simulink model "allmodes_group11"  (R2023a)
settings: Solver=FixedStepAuto  StartTime=0.0  StopTime=10.0  FixedStep=1e-3  RelTol=1e-3  EnableMultiTasking=on
undefined symbols (not defined in the file): a, A0, A1, b, c, D0, D1, D10, D11, D12, D13, D2, D3, D4, D5, D6, D7, D8, D9, magnitude, PTA0, PTA1, PTA2, PTB2, PTB23, PTB3, PTB9, PTC16, PTC17, PTC2, PTC3, PTC4, PTD0, PTD1, PTD2, PTD3
libraries: etargetslib x22, frdmk64flib x19, simulink x2, hdlsllib x1, dspstat3 x1
settings Model: ExtModeTrigDuration=5  Creator=faraa  LastModifiedBy=faraa
settings OptimizationCC: EnhancedBackFolding=on  PassReuseOutputArgsAs=Individual arguments  ZeroExternalMemoryAtStartup=off  ZeroInternalMemoryAtStartup=off  MaxStackSize=64  OptimizeBlockOrder=speed  DifferentSizesBufferReuse=on  OptimizationCustomize=off  EfficientTunableParamExpr=on
settings DebuggingCC: ParameterTunabilityLossMsg=error
settings HardwareCC: ProdBitPerPointer=32  ProdBitPerSizeT=32  ProdBitPerPtrDiffT=32  ProdLargestAtomicInteger=Long  ProdLargestAtomicFloat=Double  ProdWordSize=32  ProdHWDeviceType=ARM Compatible->ARM Cortex
settings SFSimCC: MATLABDynamicMemAlloc=off
settings RTWCC: Description=Embedded Coder  SystemTargetFile=ert.tlc  HardwareBoard=NXP FRDM-K64F  TLCOptions="-aInlineSetEventsForThisBaseRateFcn=TLC_FALSE -aSuppressMultiTaskScheduler=TLC_FALSE  -aRateBasedStepFcn=0"  TemplateMakefile=ert_default_tmf  Toolchain=GNU Tools for ARM Embedded Processors
settings CodeAppCC: ForceParamTrailComments=on  IgnoreCustomStorageClasses=off  OperatorAnnotations=on  SimulinkDataObjDesc=on  SFDataObjDesc=on  InsertBlockDesc=on
settings ERTTargetCC: ExtModeTransport=4  ExtModeMexFile=sendToCommService

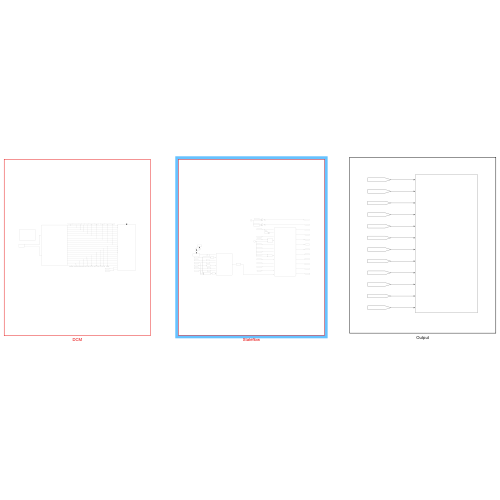
[thumbnail: Simulink's stored preview of the top-level diagram]
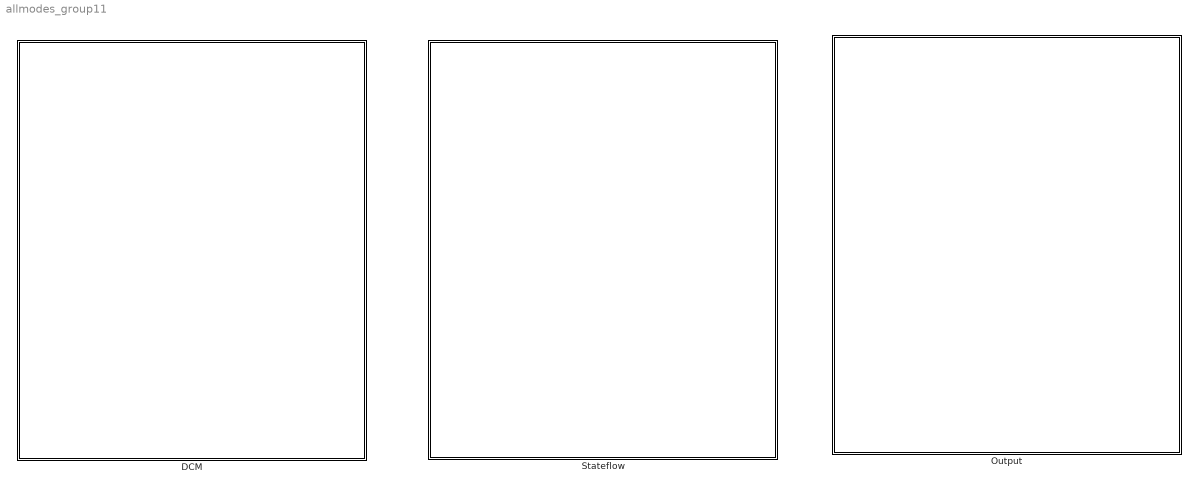
== system allmodes_group11 ==
  DCM : Subsystem
  Output : Subsystem
  Stateflow : Subsystem

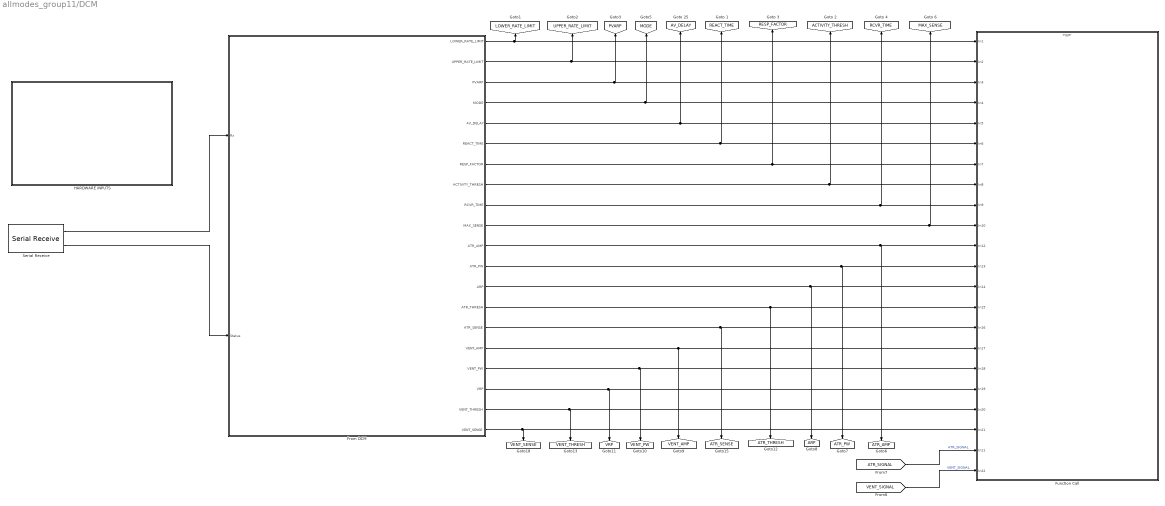
== system allmodes_group11/DCM ==
  From DCM : Stateflow chart  TreatAsAtomicUnit=on
  Function Call : Subsystem  TreatAsAtomicUnit=on
  HARDWARE INPUTS : Subsystem
  Serial Receive : frdmk64flib/Serial Receive  SCIModule=0  Baudrate=uint32(9600)  Parity=None  StopBits=1  HardwareFlowControl=None  ByteOrder=LittleEndian  DataType=uint8  DataLength=86  BlockingMode=off  OutputStatus=on  SampleTime=-1
  tag scope: ACTIVITY_THRESH=global, ARP=global, ATR_AMP=global, ATR_PW=global, ATR_SENSE=global, ATR_THRESH=global, AV_DELAY=global, LOWER_RATE_LIMIT=global, MAX_SENSE=global, MODE=global, PVARP=global, RCVR_TIME=global, REACT_TIME=global, RESP_FACTOR=global, UPPER_RATE_LIMIT=global, VENT_AMP=global, VENT_PW=global, VENT_SENSE=global, VENT_THRESH=global, VRP=global
  wires:
  Serial Receive/1 -> From DCM/1(Rx)
  Serial Receive/2 -> From DCM/2(Status)
  From DCM/1(LOWER_RATE_LIMIT) -> Function Call/1(In1), [LOWER_RATE_LIMIT]
  From DCM/2(UPPER_RATE_LIMIT) -> Function Call/2(In2), [UPPER_RATE_LIMIT]
  From DCM/3(PVARP) -> [PVARP], Function Call/3(In3)
  From DCM/4(MODE) -> Function Call/4(In4), [MODE]
  From DCM/5(AV_DELAY) -> [AV_DELAY], Function Call/5(In5)
  From DCM/6(REACT_TIME) -> Function Call/6(In6), [REACT_TIME]
  From DCM/7(RESP_FACTOR) -> [RESP_FACTOR], Function Call/7(In7)
  From DCM/8(ACTIVITY_THRESH) -> [ACTIVITY_THRESH], Function Call/8(In8)
  From DCM/9(RCVR_TIME) -> [RCVR_TIME], Function Call/9(In9)
  From DCM/10(MAX_SENSE) -> [MAX_SENSE], Function Call/10(In10)
  From DCM/11(ATR_AMP) -> Function Call/11(In12), [ATR_AMP]
  From DCM/12(ATR_PW) -> Function Call/12(In13), [ATR_PW]
  From DCM/13(ARP) -> Function Call/13(In14), [ARP]
  From DCM/14(ATR_THRESH) -> Function Call/14(In15), [ATR_THRESH]
  From DCM/15(ATR_SENSE) -> Function Call/15(In16), [ATR_SENSE]
  From DCM/16(VENT_AMP) -> Function Call/16(In17), [VENT_AMP]
  From DCM/17(VENT_PW) -> Function Call/17(In18), [VENT_PW]
  From DCM/18(VRP) -> Function Call/18(In19), [VRP]
  From DCM/19(VENT_THRESH) -> Function Call/19(In20), [VENT_THRESH]
  From DCM/20(VENT_SENSE) -> Function Call/20(In21), [VENT_SENSE]
  [ATR_SIGNAL] -> Function Call/21(In11)  "ATR_SIGNAL"
  [VENT_SIGNAL] -> Function Call/22(In22)  "VENT_SIGNAL"

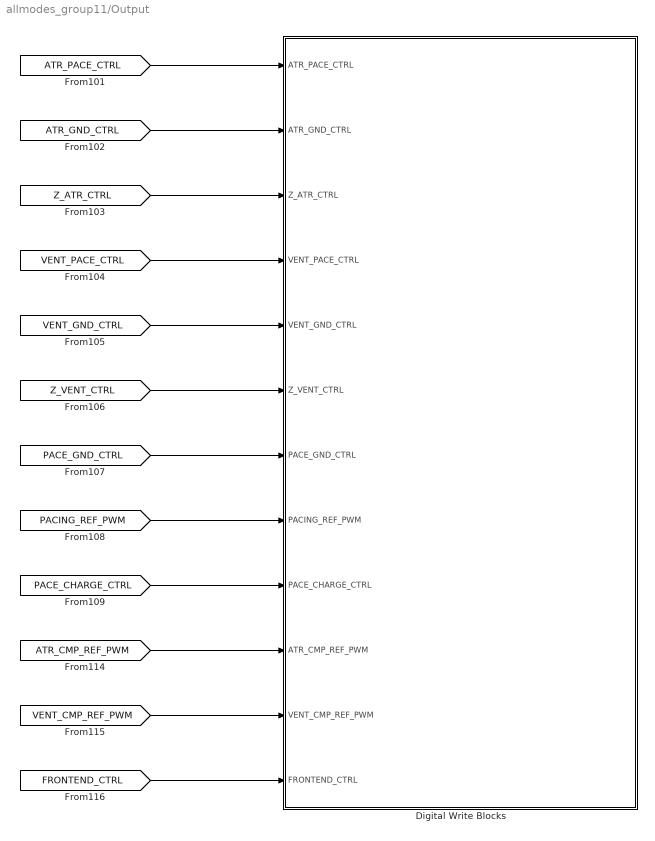
== system allmodes_group11/Output ==
  Digital Write Blocks : Subsystem
  wires:
  [Z_VENT_CTRL] -> Digital Write Blocks/6(Z_VENT_CTRL)
  [PACE_GND_CTRL] -> Digital Write Blocks/7(PACE_GND_CTRL)
  [ATR_PACE_CTRL] -> Digital Write Blocks/1(ATR_PACE_CTRL)
  [PACING_REF_PWM] -> Digital Write Blocks/8(PACING_REF_PWM)
  [VENT_GND_CTRL] -> Digital Write Blocks/5(VENT_GND_CTRL)
  [VENT_CMP_REF_PWM] -> Digital Write Blocks/11(VENT_CMP_REF_PWM)
  [PACE_CHARGE_CTRL] -> Digital Write Blocks/9(PACE_CHARGE_CTRL)
  [ATR_GND_CTRL] -> Digital Write Blocks/2(ATR_GND_CTRL)
  [VENT_PACE_CTRL] -> Digital Write Blocks/4(VENT_PACE_CTRL)
  [ATR_CMP_REF_PWM] -> Digital Write Blocks/10(ATR_CMP_REF_PWM)
  [Z_ATR_CTRL] -> Digital Write Blocks/3(Z_ATR_CTRL)
  [FRONTEND_CTRL] -> Digital Write Blocks/12(FRONTEND_CTRL)

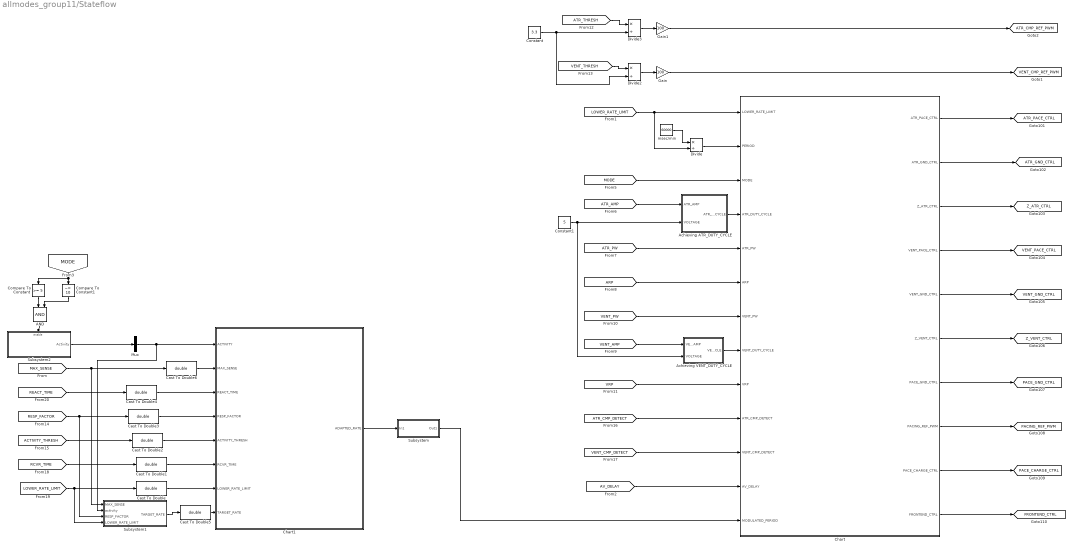
== system allmodes_group11/Stateflow ==
  AND : Logic  IconShape=distinctive  AllPortsSameDT=off  OutDataTypeStr=boolean
  Achieving ATR_DUTY_CYCLE : Subsystem
  Achieving VENT_DUTY_CYCLE : Subsystem
  Cast To Double{,1..6} (7 alike) : DataTypeConversion  OutDataTypeStr=double  SaturateOnIntegerOverflow=off  RndMeth=Floor
  Chart : Stateflow chart  TreatAsAtomicUnit=on
  Chart1 : Stateflow chart  TreatAsAtomicUnit=on
  Compare To Constant : simulink/Logic and Bit Operations/Compare To Constant  relop=>=  const=5  OutDataTypeStr=boolean
  Compare To Constant1 : simulink/Logic and Bit Operations/Compare To Constant  relop=~=  const=10  OutDataTypeStr=boolean
  Constant : Constant  Value=3.3
  Constant1 : Constant  Value=5
  Divide : Product  Inputs=*/
  Divide2 : Product  Inputs=*/
  Divide3 : Product  Inputs=*/
  Gain : Gain  Gain=100
  Gain1 : Gain  Gain=100
  Mux : Mux  Inputs=1
  Subsystem : Subsystem
  Subsystem1 : Subsystem
  Subsystem2 : Subsystem
  msec/min : Constant  Value=60000  OutDataTypeStr=double  LockScale=on
  tag scope: ATR_CMP_REF_PWM=global, ATR_GND_CTRL=global, ATR_PACE_CTRL=global, FRONTEND_CTRL=global, PACE_CHARGE_CTRL=global, PACE_GND_CTRL=global, PACING_REF_PWM=global, VENT_CMP_REF_PWM=global, VENT_GND_CTRL=global, VENT_PACE_CTRL=global, Z_ATR_CTRL=global, Z_VENT_CTRL=global
  wires:
  [VRP] -> Chart/9(VRP)
  [MODE] -> Chart/3(MODE)
  [LOWER_RATE_LIMIT] -> Divide/2, Chart/1(LOWER_RATE_LIMIT)
  [ATR_PW] -> Chart/5(ATR_PW)
  [ARP] -> Chart/6(ARP)
  [ATR_AMP] -> Achieving ATR_DUTY_CYCLE/1(ATR_AMP)
  Achieving ATR_DUTY_CYCLE/1(ATR_DUTY_CYCLE) -> Chart/4(ATR_DUTY_CYCLE)
  [VENT_PW] -> Chart/7(VENT_PW)
  [VENT_AMP] -> Achieving VENT_DUTY_CYCLE/1(VENT_AMP)
  Achieving VENT_DUTY_CYCLE/1(VENT_DUTY_CYCLE) -> Chart/8(VENT_DUTY_CYCLE)
  Chart/1(ATR_PACE_CTRL) -> [ATR_PACE_CTRL]
  Chart/2(ATR_GND_CTRL) -> [ATR_GND_CTRL]
  Chart/3(Z_ATR_CTRL) -> [Z_ATR_CTRL]
  Chart/4(VENT_PACE_CTRL) -> [VENT_PACE_CTRL]
  Chart/5(VENT_GND_CTRL) -> [VENT_GND_CTRL]
  Chart/6(Z_VENT_CTRL) -> [Z_VENT_CTRL]
  Chart/7(PACE_GND_CTRL) -> [PACE_GND_CTRL]
  Chart/8(PACING_REF_PWM) -> [PACING_REF_PWM]
  Chart/9(PACE_CHARGE_CTRL) -> [PACE_CHARGE_CTRL]
  Constant1/1 -> Achieving VENT_DUTY_CYCLE/2(VOLTAGE), Achieving ATR_DUTY_CYCLE/2(VOLTAGE)
  [ATR_CMP_DETECT] -> Chart/10(ATR_CMP_DETECT)
  [VENT_CMP_DETECT] -> Chart/11(VENT_CMP_DETECT)
  Divide/1 -> Chart/2(PERIOD)
  msec/min/1 -> Divide/1
  Chart/10(FRONTEND_CTRL) -> [FRONTEND_CTRL]
  Constant/1 -> Divide3/2, Divide2/2
  [ATR_THRESH] -> Divide3/1
  [VENT_THRESH] -> Divide2/1
  [AV_DELAY] -> Chart/12(AV_DELAY)
  Divide2/1 -> Gain/1
  Gain/1 -> [VENT_CMP_REF_PWM]
  Divide3/1 -> Gain1/1
  Gain1/1 -> [ATR_CMP_REF_PWM]
  [REACT_TIME] -> Cast To Double4/1
  [ACTIVITY_THRESH] -> Cast To Double2/1
  [LOWER_RATE_LIMIT] -> Cast To Double/1, Subsystem1/4(LOWER_RATE_LIMIT)
  [RCVR_TIME] -> Cast To Double1/1
  [MAX_SENSE] -> Cast To Double6/1, Subsystem1/1(MAX_SENSE)
  [MODE] -> Compare To Constant/1, Compare To Constant1/1
  [RESP_FACTOR] -> Subsystem1/3(RESP_FACTOR), Cast To Double3/1
  Subsystem2/1(Activity) -> Mux/1
  Subsystem/1(Out1) -> Chart/13(MODULATED_PERIOD)
  Compare To Constant/1 -> AND/1
  AND/1 -> Subsystem2/Enable
  Compare To Constant1/1 -> AND/2
  Subsystem1/1(TARGET_RATE) -> Cast To Double5/1
  Chart1/1(ADAPTED_RATE) -> Subsystem/1(In1)
  Mux/1 -> Subsystem1/2(activity), Chart1/1(ACTIVITY)
  Cast To Double/1 -> Chart1/7(LOWER_RATE_LIMIT)
  Cast To Double1/1 -> Chart1/6(RCVR_TIME)
  Cast To Double2/1 -> Chart1/5(ACTIVITY_THRESH)
  Cast To Double3/1 -> Chart1/4(RESP_FACTOR)
  Cast To Double4/1 -> Chart1/3(REACT_TIME)
  Cast To Double5/1 -> Chart1/8(TARGET_RATE)
  Cast To Double6/1 -> Chart1/2(MAX_SENSE)

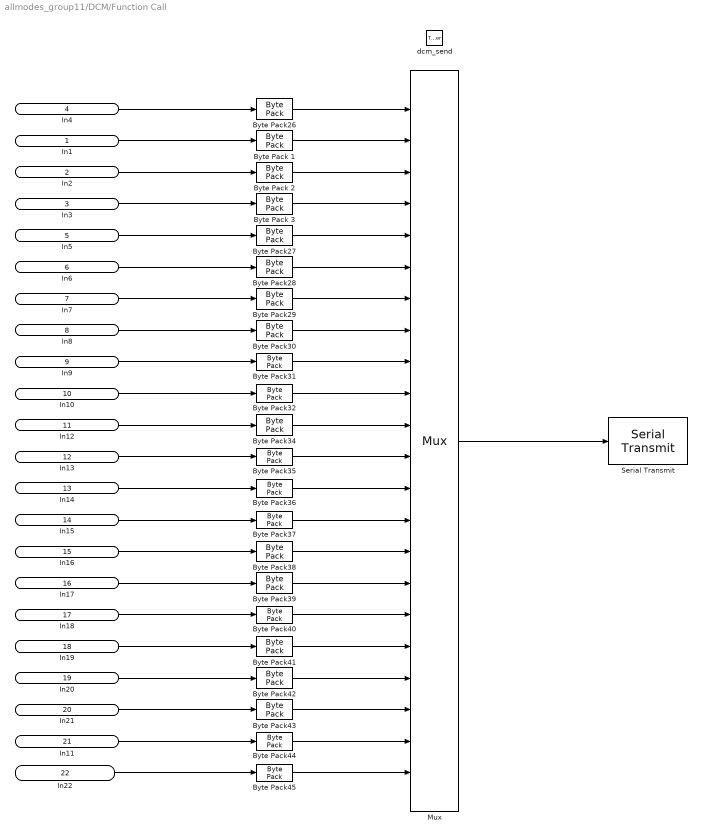
== system allmodes_group11/DCM/Function Call ==
  In1 : Inport
  In2 : Inport  Port=2
  In3 : Inport  Port=3
  In4 : Inport  Port=4
  In5 : Inport  Port=5
  In6 : Inport  Port=6
  In7 : Inport  Port=7
  In8 : Inport  Port=8
  In9 : Inport  Port=9
  In10 : Inport  Port=10
  In12 : Inport  Port=11
  In13 : Inport  Port=12
  In14 : Inport  Port=13
  In15 : Inport  Port=14
  In16 : Inport  Port=15
  In17 : Inport  Port=16
  In18 : Inport  Port=17
  In19 : Inport  Port=18
  In20 : Inport  Port=19
  In21 : Inport  Port=20
  In11 : Inport  Port=21
  In22 : Inport  Port=22
  dcm_send : TriggerPort  TriggerType=function-call  IsSimulinkFunction=on  FunctionName=dcm_send  VariantControl=Variant
  Byte Pack 1 : etargetslib/Byte Pack  datatypes={'uint16'}  byteAlign=1
  Byte Pack 2 : etargetslib/Byte Pack  datatypes={'uint16'}  byteAlign=1
  Byte Pack 3 : etargetslib/Byte Pack  datatypes={'uint16'}  byteAlign=1
  Byte Pack{26..29,31..32,35..36,40..41} (10 alike) : etargetslib/Byte Pack  datatypes={'uint16'}  byteAlign=1
  Byte Pack{30,34,37..39,42..45} (9 alike) : etargetslib/Byte Pack  datatypes={'double'}  byteAlign=1
  Mux : Mux  Inputs=22
  Serial Transmit : frdmk64flib/Serial Transmit  SCIModule=0  Baudrate=uint32(9600)  Parity=None  StopBits=1  HardwareFlowControl=None  ByteOrder=LittleEndian  BlockingMode=on  OutputStatus=on
  wires:
  In1/1 -> Byte Pack 1/1
  In2/1 -> Byte Pack 2/1
  In3/1 -> Byte Pack 3/1
  In4/1 -> Byte Pack26/1
  In5/1 -> Byte Pack27/1
  In6/1 -> Byte Pack28/1
  In7/1 -> Byte Pack29/1
  In8/1 -> Byte Pack30/1
  In9/1 -> Byte Pack31/1
  In10/1 -> Byte Pack32/1
  In12/1 -> Byte Pack34/1
  In13/1 -> Byte Pack35/1
  In14/1 -> Byte Pack36/1
  In15/1 -> Byte Pack37/1
  In16/1 -> Byte Pack38/1
  In17/1 -> Byte Pack39/1
  In18/1 -> Byte Pack40/1
  In19/1 -> Byte Pack41/1
  In20/1 -> Byte Pack42/1
  In21/1 -> Byte Pack43/1
  Byte Pack27/1 -> Mux/5
  Byte Pack28/1 -> Mux/6
  Byte Pack29/1 -> Mux/7
  Byte Pack30/1 -> Mux/8
  Byte Pack31/1 -> Mux/9
  Byte Pack32/1 -> Mux/10
  Byte Pack34/1 -> Mux/11
  Byte Pack35/1 -> Mux/12
  Byte Pack36/1 -> Mux/13
  Byte Pack37/1 -> Mux/14
  Byte Pack38/1 -> Mux/15
  Byte Pack39/1 -> Mux/16
  Byte Pack40/1 -> Mux/17
  Byte Pack41/1 -> Mux/18
  Byte Pack42/1 -> Mux/19
  Byte Pack43/1 -> Mux/20
  Mux/1 -> Serial Transmit/1
  Byte Pack44/1 -> Mux/21
  Byte Pack45/1 -> Mux/22
  Byte Pack26/1 -> Mux/1
  Byte Pack 1/1 -> Mux/2
  Byte Pack 2/1 -> Mux/3
  Byte Pack 3/1 -> Mux/4
  In22/1 -> Byte Pack45/1
  In11/1 -> Byte Pack44/1

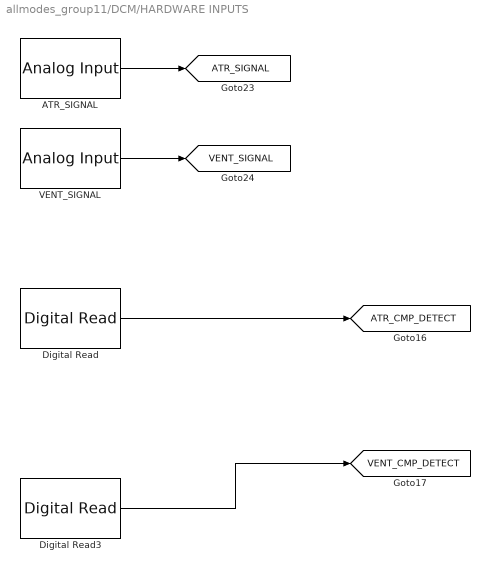
== system allmodes_group11/DCM/HARDWARE INPUTS ==
  ATR_SIGNAL : frdmk64flib/Analog Input  Whichpin=PTB2 (A0)  SampleTime=-1
  Digital Read : frdmk64flib/Digital Read  Whichpin=PTC16 (D0)  SampleTime=-1
  Digital Read3 : frdmk64flib/Digital Read  Whichpin=PTC17 (D1)  SampleTime=-1
  VENT_SIGNAL : frdmk64flib/Analog Input  Whichpin=PTB3 (A1)  SampleTime=-1
  tag scope: ATR_CMP_DETECT=global, ATR_SIGNAL=global, VENT_CMP_DETECT=global, VENT_SIGNAL=global
  wires:
  VENT_SIGNAL/1 -> [VENT_SIGNAL]
  ATR_SIGNAL/1 -> [ATR_SIGNAL]
  Digital Read3/1 -> [VENT_CMP_DETECT]
  Digital Read/1 -> [ATR_CMP_DETECT]

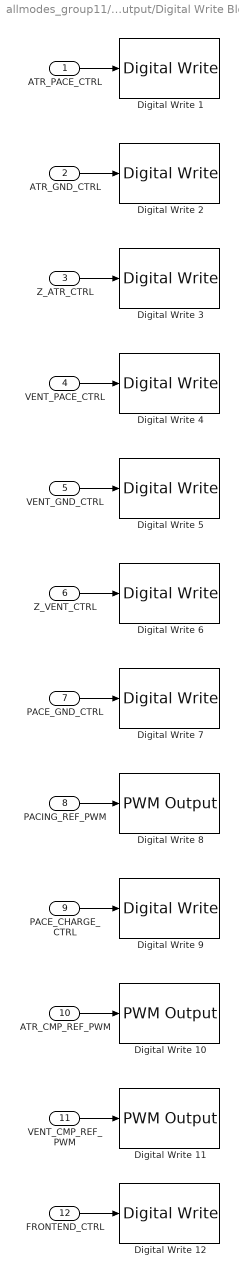
== system allmodes_group11/Output/Digital Write Blocks ==
  ATR_PACE_CTRL : Inport
  ATR_GND_CTRL : Inport  Port=2
  Z_ATR_CTRL : Inport  Port=3
  VENT_PACE_CTRL : Inport  Port=4
  VENT_GND_CTRL : Inport  Port=5
  Z_VENT_CTRL : Inport  Port=6
  PACE_GND_CTRL : Inport  Port=7
  PACING_REF_PWM : Inport  Port=8
  PACE_CHARGE_CTRL : Inport  Port=9
  ATR_CMP_REF_PWM : Inport  Port=10
  VENT_CMP_REF_PWM : Inport  Port=11  OutDataTypeStr=double
  FRONTEND_CTRL : Inport  Port=12
  Digital Write 1 : frdmk64flib/Digital Write  Whichpin=PTA0 (D8)
  Digital Write 10 : frdmk64flib/PWM Output  Whichpin=PTC2 (D6)  InitialFrequency=2000  InitialDutyCycle=30
  Digital Write 11 : frdmk64flib/PWM Output  Whichpin=PTA1 (D3)  InitialFrequency=2000  InitialDutyCycle=30
  Digital Write 12 : frdmk64flib/Digital Write  Whichpin=PTD1 (D13)
  Digital Write 2 : frdmk64flib/Digital Write  Whichpin=PTD2 (D11)
  Digital Write 3 : frdmk64flib/Digital Write  Whichpin=PTB23 (D4)
  Digital Write 4 : frdmk64flib/Digital Write  Whichpin=PTC4 (D9)
  Digital Write 5 : frdmk64flib/Digital Write  Whichpin=PTD3 (D12)
  Digital Write 6 : frdmk64flib/Digital Write  Whichpin=PTC3 (D7)
  Digital Write 7 : frdmk64flib/Digital Write  Whichpin=PTD0 (D10)
  Digital Write 8 : frdmk64flib/PWM Output  Whichpin=PTA2 (D5)  InitialFrequency=2000  InitialDutyCycle=30
  Digital Write 9 : frdmk64flib/Digital Write  Whichpin=PTB9 (D2)
  wires:
  VENT_PACE_CTRL/1 -> Digital Write 4/1
  VENT_GND_CTRL/1 -> Digital Write 5/1
  ATR_GND_CTRL/1 -> Digital Write 2/1
  PACING_REF_PWM/1 -> Digital Write 8/1
  ATR_PACE_CTRL/1 -> Digital Write 1/1
  PACE_GND_CTRL/1 -> Digital Write 7/1
  Z_VENT_CTRL/1 -> Digital Write 6/1
  PACE_CHARGE_CTRL/1 -> Digital Write 9/1
  Z_ATR_CTRL/1 -> Digital Write 3/1
  ATR_CMP_REF_PWM/1 -> Digital Write 10/1
  VENT_CMP_REF_PWM/1 -> Digital Write 11/1
  FRONTEND_CTRL/1 -> Digital Write 12/1

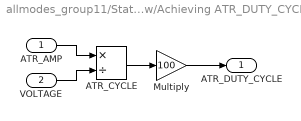
== system allmodes_group11/Stateflow/Achieving ATR_DUTY_CYCLE ==
  ATR_AMP : Inport
  VOLTAGE : Inport  Port=2
  ATR_CYCLE : Product  Inputs=*/
  Multiply : Gain  Gain=100
  ATR_DUTY_CYCLE : Outport  VectorParamsAs1DForOutWhenUnconnected=off
  wires:
  ATR_AMP/1 -> ATR_CYCLE/1
  VOLTAGE/1 -> ATR_CYCLE/2
  ATR_CYCLE/1 -> Multiply/1
  Multiply/1 -> ATR_DUTY_CYCLE/1

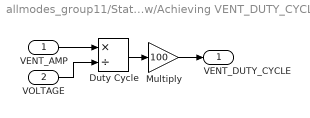
== system allmodes_group11/Stateflow/Achieving VENT_DUTY_CYCLE ==
  VENT_AMP : Inport
  VOLTAGE : Inport  Port=2
  Duty Cycle : Product  Inputs=*/
  Multiply : Gain  Gain=100
  VENT_DUTY_CYCLE : Outport  VectorParamsAs1DForOutWhenUnconnected=off
  wires:
  VENT_AMP/1 -> Duty Cycle/1
  VOLTAGE/1 -> Duty Cycle/2
  Duty Cycle/1 -> Multiply/1
  Multiply/1 -> VENT_DUTY_CYCLE/1

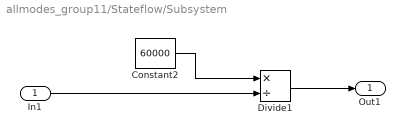
== system allmodes_group11/Stateflow/Subsystem ==
  In1 : Inport
  Constant2 : Constant  Value=60000
  Divide1 : Product  Inputs=*/
  Out1 : Outport
  wires:
  In1/1 -> Divide1/2
  Constant2/1 -> Divide1/1
  Divide1/1 -> Out1/1

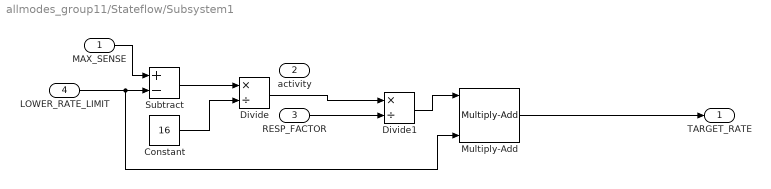
== system allmodes_group11/Stateflow/Subsystem1 ==
  MAX_SENSE : Inport
  activity : Inport  Port=2
  RESP_FACTOR : Inport  Port=3
  LOWER_RATE_LIMIT : Inport  Port=4
  Constant : Constant  Value=16
  Divide : Product  Inputs=*/
  Divide1 : Product  Inputs=*/
  Multiply-Add : hdlsllib/HDL Operations/Multiply-Add  Function=c+(a.*b)  datatype=uint16  RndMeth=Nearest  DoSatur=off  FMA=off
  Subtract : Sum  Inputs=+-
  TARGET_RATE : Outport  OutDataTypeStr=uint16  SourceOfInitialOutputValue=Input signal
  wires:
  MAX_SENSE/1 -> Subtract/1
  LOWER_RATE_LIMIT/1 -> Multiply-Add/3, Subtract/2
  Subtract/1 -> Divide/1
  Constant/1 -> Divide/2
  Divide/1 -> Divide1/1
  RESP_FACTOR/1 -> Divide1/2
  Divide1/1 -> Multiply-Add/1
  Multiply-Add/1 -> TARGET_RATE/1

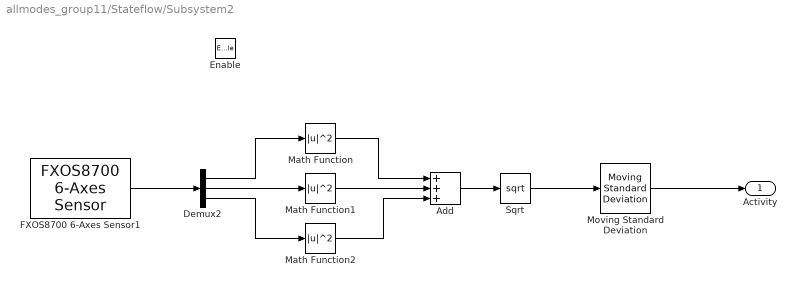
== system allmodes_group11/Stateflow/Subsystem2 ==
  Enable : EnablePort
  Add : Sum  Inputs=+++
  Demux2 : Demux  Outputs=3
  FXOS8700 6-Axes Sensor1 : frdmk64flib/FXOS8700 6-Axes Sensor  Activesensor=Accelerometer only  ODR=800Hz  HybridODR=400Hz  Accelfullrange=-4g to +4g  SampleTime=-1
  Math Function : Math  Operator=magnitude^2  SignedPower=on  OutDataTypeStr=double
  Math Function1 : Math  Operator=magnitude^2  SignedPower=on  OutDataTypeStr=double
  Math Function2 : Math  Operator=magnitude^2  SignedPower=on  OutDataTypeStr=double
  Moving Standard Deviation : dspstat3/Moving Standard Deviation  Method=Sliding window  ForgettingFactorPort=off  SpecifyWindowLength=on  WindowLength=128  OverlapLength=127  AllowArbitraryInputLength=off  ForgettingFactor=0.9  SimulateUsing=Code generation
  Sqrt : Sqrt
  Activity : Outport  SourceOfInitialOutputValue=Input signal
  wires:
  Sqrt/1 -> Moving Standard Deviation/1
  FXOS8700 6-Axes Sensor1/1 -> Demux2/1
  Math Function/1 -> Add/1
  Add/1 -> Sqrt/1
  Math Function2/1 -> Add/3
  Demux2/2 -> Math Function1/1
  Math Function1/1 -> Add/2
  Demux2/1 -> Math Function/1
  Demux2/3 -> Math Function2/1
  Moving Standard Deviation/1 -> Activity/1

== stateflow chart allmodes_group11/DCM/From DCM ==
  state ECHO_PARAM2
    entry:
    dcm_send();
  state Default
    %Setting values to variables if
    %not initialized in DCM
    entry:
    %GENERAL
    MODE = 7;
    LOWER_RATE_LIMIT = 60;
    UPPER_RATE_LIMIT = 120;
    PVARP = 250;
    AV_DELAY = 150;
    REACT_TIME = 50;
    RESP_FACTOR = 16;
    ACTIVITY_THRESH = 0.2;
    RCVR_TIME = 60;
    MAX_SENSE = 180;
    %ATRIUM
    ATR_AMP = 600;
    ATR_PW = 10;
    ARP = 200;
    ATR_THRESH = 1.8;
    ATR_SENSE = 800;
    %VENTRICLE
    VENT_AMP = 600;
    VENT_PW = 10;
    VRP = 200;
    VENT_THRESH = 2.2;
    VENT_SENSE = 800;
  state SET_PARAM
    entry:
    MODE = typecast(Rx(3:4), 'uint16');
    LOWER_RATE_LIMIT = typecast(Rx(5:6), 'uint16');
    UPPER_RATE_LIMIT = typecast(Rx(7:8), 'uint16');
    PVARP = typecast(Rx(9:10), 'uint16');
    AV_DELAY = typecast(Rx(11:12), 'uint16');
    REACT_TIME = typecast(Rx(13:14), 'uint16');
    RESP_FACTOR = typecast(Rx(15:16), 'uint16');
    ACTIVITY_THRESH = typecast(Rx(17:24), 'double');
    RCVR_TIME = typecast(Rx(25:26), 'uint16');
    MAX_SENSE = typecast(Rx(27:28), 'uint16');
    %ATR
    ATR_AMP = typecast(Rx(29:36), 'double');
    ATR_PW = typecast(Rx(37:38), 'uint16');
    ARP = typecast(Rx(39:40), 'uint16');
    ATR_THRESH = typecast(Rx(41:48), 'double');
    ATR_SENSE = typecast(Rx(49:56), 'double');
    %VENT
    VENT_AMP = typecast(Rx(57:64), 'double');
    VENT_PW = typecast(Rx(65:66), 'uint16');
    VRP = typecast(Rx(67:68), 'uint16');
    VENT_THRESH = typecast(Rx(69:76), 'double');
    VENT_SENSE = typecast(Rx(77:84), 'double');
  state STANDBY
  state ECHO_PARAM
    entry:
    dcm_send();
  ECHO_PARAM2 -> STANDBY
  SET_PARAM -> ECHO_PARAM2
  (default) -> Default
  (junction 7) -> STANDBY [order 2]
  Default -> STANDBY
  STANDBY -> (junction 7) : [Status == 0]
  (junction 7) -> (junction 10) [order 1] : [Rx(1) == hex2dec('00')]
  (junction 10) -> SET_PARAM [order 2] : [Rx(2) == hex2dec('00')]
  (junction 10) -> ECHO_PARAM [order 1] : [Rx(2) == hex2dec('01')]
  ECHO_PARAM -> STANDBY
  data: Rx input uint8; Status input uint8; LOWER_RATE_LIMIT output uint16; UPPER_RATE_LIMIT output uint16; PVARP output uint16; MODE output uint16; AV_DELAY output uint16; REACT_TIME output uint16; RESP_FACTOR output uint16; ACTIVITY_THRESH output double; RCVR_TIME output uint16; MAX_SENSE output uint16; ATR_AMP output double; ATR_PW output uint16; ARP output uint16; ATR_THRESH output double; ATR_SENSE output double; VENT_AMP output double; VENT_PW output uint16; VRP output uint16; VENT_THRESH output double; VENT_SENSE output double

== stateflow chart allmodes_group11/Stateflow/Chart ==
  state Start
  state AOO [group]
    state CHARGING
      during:
      %Begin Charging C22 Capacitor
      ATR_PACE_CTRL = LOW
      VENT_PACE_CTRL = LOW
      PACING_REF_PWM = ATR_DUTY_CYCLE
      PACE_CHARGE_CTRL = HIGH
      %Begin Discharging C21 Blocking Capacitor
      PACE_GND_CTRL = HIGH
      VENT_PACE_CTRL = LOW
      Z_ATR_CTRL = LOW
      Z_VENT_CTRL = LOW
      ATR_PACE_CTRL = LOW
      ATR_GND_CTRL = HIGH
      VENT_GND_CTRL = LOW
    state DISCHARGING
      during:
      %Discharge C22 into Atrium (AtrialPacing)
      %Begin Charging C21 Blocking Capacitor
      PACE_CHARGE_CTRL = LOW
      PACE_GND_CTRL = HIGH
      ATR_PACE_CTRL = HIGH
      ATR_GND_CTRL = LOW
      Z_ATR_CTRL = LOW
      Z_VENT_CTRL = LOW
      VENT_GND_CTRL = LOW
      VENT_PACE_CTRL  = LOW
    AOO.CHARGING -> AOO.DISCHARGING [order 1] : after(PERIOD-ATR_PW, msec)
    AOO.DISCHARGING -> AOO.CHARGING : after(ATR_PW, msec)
  state AAI [group]
    state PROXY
      during:
      %Discharge C21 Blocking Capacitor
      PACE_GND_CTRL = HIGH
      VENT_PACE_CTRL = LOW
      Z_ATR_CTRL = LOW
      Z_VENT_CTRL = LOW
      ATR_PACE_CTRL = LOW
      ATR_GND_CTRL = HIGH
      VENT_GND_CTRL = LOW
      %Charge C22
      ATR_PACE_CTRL = LOW
      VENT_PACE_CTRL = LOW
      PACING_REF_PWM = ATR_DUTY_CYCLE
      PACE_CHARGE_CTRL = HIGH
    state DISCHARGING
      during:
      %Discharge C22 into Atrium (Atrial Pacing)
      %Begin Charging Blocking Capacitor
      PACE_CHARGE_CTRL = LOW
      PACE_GND_CTRL = HIGH
      ATR_PACE_CTRL = HIGH
      ATR_GND_CTRL = LOW
      Z_ATR_CTRL = LOW
      Z_VENT_CTRL = LOW
      VENT_GND_CTRL = LOW
      VENT_PACE_CTRL  = LOW
    state CHARGING
      during:
      %Begin Charging C22 Capacitor
      ATR_PACE_CTRL = LOW
      VENT_PACE_CTRL = LOW
      PACING_REF_PWM = ATR_DUTY_CYCLE
      PACE_CHARGE_CTRL = HIGH
      %Begin Discharging C21 Blocking Capacitor
      PACE_GND_CTRL = HIGH
      VENT_PACE_CTRL = LOW
      Z_ATR_CTRL = LOW
      Z_VENT_CTRL = LOW
      ATR_PACE_CTRL = LOW
      ATR_GND_CTRL = HIGH
      VENT_GND_CTRL = LOW
    AAI.DISCHARGING -> AAI.PROXY : after(ATR_PW,msec)
    AAI.PROXY -> AAI.CHARGING : after(ARP, msec)
    (junction 116) -> AAI.PROXY : after(LOWER_RATE_LIMIT,msec)
    AAI.CHARGING -> (junction 116) [order 1] : [ATR_CMP_DETECT == HIGH]
    AAI.CHARGING -> AAI.DISCHARGING [order 2] : after(PERIOD-ATR_PW-ARP,msec)
  state VOO [group]
    state CHARGING
      during:
      %Begin Charging C22 Capacitor
      ATR_PACE_CTRL = LOW
      VENT_PACE_CTRL = LOW
      PACING_REF_PWM = VENT_DUTY_CYCLE
      PACE_CHARGE_CTRL = HIGH
      %Begin Discharging C21 Blocking Capacitor
      PACE_GND_CTRL = HIGH
      VENT_PACE_CTRL = LOW
      Z_ATR_CTRL = LOW
      Z_VENT_CTRL = LOW
      ATR_PACE_CTRL = LOW
      ATR_GND_CTRL = LOW
      VENT_GND_CTRL = HIGH
    state DISCHARGING
      during:
      %Discharge C22 into Ventricle (Vent Pacing)
      %Begin Charging Blocking Capacitor
      PACE_CHARGE_CTRL = LOW
      PACE_GND_CTRL = HIGH
      ATR_PACE_CTRL = LOW
      ATR_GND_CTRL = LOW
      Z_ATR_CTRL = LOW
      Z_VENT_CTRL = LOW
      VENT_GND_CTRL = LOW
      VENT_PACE_CTRL  = HIGH
    VOO.CHARGING -> VOO.DISCHARGING [order 1] : after(PERIOD-VENT_PW,msec)
    VOO.DISCHARGING -> VOO.CHARGING : after(VENT_PW,msec)
  state VVI [group]
    state PROXY
      during:
      %Step 1
      %Discharge C21 Blocking Capacitor
      PACE_GND_CTRL = HIGH
      VENT_PACE_CTRL = LOW
      Z_ATR_CTRL = LOW
      Z_VENT_CTRL = LOW
      ATR_PACE_CTRL = LOW
      ATR_GND_CTRL = LOW
      VENT_GND_CTRL = HIGH
      %Step 2
      %Charge C22
      ATR_PACE_CTRL = LOW
      VENT_PACE_CTRL = LOW
      PACING_REF_PWM = VENT_DUTY_CYCLE
      PACE_CHARGE_CTRL = HIGH
    state CHARGING
      during:
      %Begin Charging C22 Capacitor
      ATR_PACE_CTRL = LOW
      VENT_PACE_CTRL = LOW
      PACING_REF_PWM = VENT_DUTY_CYCLE
      PACE_CHARGE_CTRL = HIGH
      %Begin Discharging Blocking Capacitor
      PACE_GND_CTRL = HIGH
      VENT_PACE_CTRL = LOW
      Z_ATR_CTRL = LOW
      Z_VENT_CTRL = LOW
      ATR_PACE_CTRL = LOW
      ATR_GND_CTRL = LOW
      VENT_GND_CTRL = HIGH
    state DISCHARGING
      during:
      %Step 1:
      %Discharge C22 into Ventricle (Vent Pacing)
      %Begin Charging Blocking Capacitor
      PACE_CHARGE_CTRL = LOW
      PACE_GND_CTRL = HIGH
      ATR_PACE_CTRL = LOW
      ATR_GND_CTRL = LOW
      Z_ATR_CTRL = LOW
      Z_VENT_CTRL = LOW
      VENT_GND_CTRL = LOW
      VENT_PACE_CTRL  = HIGH
    VVI.DISCHARGING -> VVI.PROXY : after(VENT_PW, msec)
    VVI.PROXY -> VVI.CHARGING : after(VRP, msec)
    (junction 196) -> VVI.PROXY : after(LOWER_RATE_LIMIT,msec)
    VVI.CHARGING -> (junction 196) [order 1] : [VENT_CMP_DETECT ==  HIGH]
    VVI.CHARGING -> VVI.DISCHARGING [order 2] : after(PERIOD-VENT_PW-VRP,msec)
  state AOOR [group]
    state CHARGING
      during:
      %Begin Charging C22 Capacitor
      ATR_PACE_CTRL = LOW
      VENT_PACE_CTRL = LOW
      PACING_REF_PWM = ATR_DUTY_CYCLE
      PACE_CHARGE_CTRL = HIGH
      %Begin Discharging C21 Blocking Capacitor
      PACE_GND_CTRL = HIGH
      VENT_PACE_CTRL = LOW
      Z_ATR_CTRL = LOW
      Z_VENT_CTRL = LOW
      ATR_PACE_CTRL = LOW
      ATR_GND_CTRL = HIGH
      VENT_GND_CTRL = LOW
    state DISCHARGING
      during:
      %Discharge C22 into Atrium (AtrialPacing)
      %Begin Charging C21 Blocking Capacitor
      PACE_CHARGE_CTRL = LOW
      PACE_GND_CTRL = HIGH
      ATR_PACE_CTRL = HIGH
      ATR_GND_CTRL = LOW
      Z_ATR_CTRL = LOW
      Z_VENT_CTRL = LOW
      VENT_GND_CTRL = LOW
      VENT_PACE_CTRL  = LOW
    AOOR.CHARGING -> AOOR.DISCHARGING [order 1] : after(MODULATED_PERIOD - ATR_PW, msec)
    AOOR.DISCHARGING -> AOOR.CHARGING : after(ATR_PW, msec)
  state VOOR [group]
    state CHARGING
      during:
      %Begin Charging C22 Capacitor
      ATR_PACE_CTRL = LOW
      VENT_PACE_CTRL = LOW
      PACING_REF_PWM = VENT_DUTY_CYCLE
      PACE_CHARGE_CTRL = HIGH
      %Begin Discharging C21 Blocking Capacitor
      PACE_GND_CTRL = HIGH
      VENT_PACE_CTRL = LOW
      Z_ATR_CTRL = LOW
      Z_VENT_CTRL = LOW
      ATR_PACE_CTRL = LOW
      ATR_GND_CTRL = LOW
      VENT_GND_CTRL = HIGH
    state DISCHARGING
      during:
      %Discharge C22 into Ventricle (Vent Pacing)
      %Begin Charging Blocking Capacitor
      PACE_CHARGE_CTRL = LOW
      PACE_GND_CTRL = HIGH
      ATR_PACE_CTRL = LOW
      ATR_GND_CTRL = LOW
      Z_ATR_CTRL = LOW
      Z_VENT_CTRL = LOW
      VENT_GND_CTRL = LOW
      VENT_PACE_CTRL  = HIGH
    VOOR.CHARGING -> VOOR.DISCHARGING [order 1] : after(MODULATED_PERIOD - VENT_PW, msec)
    VOOR.DISCHARGING -> VOOR.CHARGING : after(VENT_PW,msec)
  state AAIR [group]
    state CHARGE_AAIR
      during:
      %Begin Charging C22 Capacitor
      ATR_PACE_CTRL = LOW;
      VENT_PACE_CTRL = LOW;
      PACING_REF_PWM = ATR_DUTY_CYCLE
      PACE_CHARGE_CTRL = HIGH;
      %Begin Discharging C21 Blocking Capacitor
      PACE_GND_CTRL = HIGH;
      VENT_PACE_CTRL = LOW;
      Z_ATR_CTRL = LOW;
      Z_VENT_CTRL = LOW;
      ATR_PACE_CTRL = LOW;
      ATR_GND_CTRL = HIGH;
      VENT_GND_CTRL = LOW;
    state PACE_AAIR
      during:
      %Discharge C22 into Atrium (Atrial Pacing)
      %Begin Charging Blocking Capacitor
      PACE_CHARGE_CTRL = LOW;
      PACE_GND_CTRL = HIGH;
      ATR_PACE_CTRL = HIGH;
      ATR_GND_CTRL = LOW;
      Z_ATR_CTRL = LOW;
      Z_VENT_CTRL = LOW;
      VENT_GND_CTRL = LOW;
      VENT_PACE_CTRL  = LOW;
    state DECIDE_AAIR
      during:
      %Discharge C21 Blocking Capacitor
      PACE_GND_CTRL = HIGH;
      VENT_PACE_CTRL = LOW;
      Z_ATR_CTRL = LOW;
      Z_VENT_CTRL = LOW;
      ATR_PACE_CTRL = LOW;
      ATR_GND_CTRL = HIGH;
      VENT_GND_CTRL = LOW;
      %Charge C22
      ATR_PACE_CTRL = LOW;
      VENT_PACE_CTRL = LOW;
      PACING_REF_PWM = ATR_DUTY_CYCLE
      PACE_CHARGE_CTRL = HIGH;
      FRONTEND_CTRL = HIGH;
    CHARGE_AAIR -> PACE_AAIR [order 2] : after(MODULATED_PERIOD - ATR_PW-ARP,msec)
    CHARGE_AAIR -> (junction 637) [order 1] : [ATR_CMP_DETECT == HIGH]
    DECIDE_AAIR -> CHARGE_AAIR : after(ARP, msec)
    PACE_AAIR -> DECIDE_AAIR : after(ATR_PW,msec)
    (junction 637) -> DECIDE_AAIR : after(LOWER_RATE_LIMIT,msec)
  state VVIR [group]
    state PROXY
      during:
      %Step 1
      %Discharge C21 Blocking Capacitor
      PACE_GND_CTRL = HIGH
      VENT_PACE_CTRL = LOW
      Z_ATR_CTRL = LOW
      Z_VENT_CTRL = LOW
      ATR_PACE_CTRL = LOW
      ATR_GND_CTRL = LOW
      VENT_GND_CTRL = HIGH
      %Step 2
      %Charge C22
      ATR_PACE_CTRL = LOW
      VENT_PACE_CTRL = LOW
      PACING_REF_PWM = VENT_DUTY_CYCLE
      PACE_CHARGE_CTRL = HIGH
    state CHARGING
      during:
      %Begin Charging C22 Capacitor
      ATR_PACE_CTRL = LOW
      VENT_PACE_CTRL = LOW
      PACING_REF_PWM = VENT_DUTY_CYCLE
      PACE_CHARGE_CTRL = HIGH
      %Begin Discharging Blocking Capacitor
      PACE_GND_CTRL = HIGH
      VENT_PACE_CTRL = LOW
      Z_ATR_CTRL = LOW
      Z_VENT_CTRL = LOW
      ATR_PACE_CTRL = LOW
      ATR_GND_CTRL = LOW
      VENT_GND_CTRL = HIGH
    state DISCHARGING
      during:
      %Step 1:
      %Discharge C22 into Ventricle (Vent Pacing)
      %Begin Charging Blocking Capacitor
      PACE_CHARGE_CTRL = LOW
      PACE_GND_CTRL = HIGH
      ATR_PACE_CTRL = LOW
      ATR_GND_CTRL = LOW
      Z_ATR_CTRL = LOW
      Z_VENT_CTRL = LOW
      VENT_GND_CTRL = LOW
      VENT_PACE_CTRL  = HIGH
    VVIR.DISCHARGING -> VVIR.PROXY : after(VENT_PW, msec)
    VVIR.PROXY -> VVIR.CHARGING : after(VRP, msec)
    (junction 451) -> VVIR.PROXY : after(LOWER_RATE_LIMIT,msec)
    VVIR.CHARGING -> (junction 451) [order 1] : [VENT_CMP_DETECT ==  HIGH]
    VVIR.CHARGING -> VVIR.DISCHARGING [order 2] : after(MODULATED_PERIOD - VENT_PW - VRP,msec)
  state DDDR [group]
    state VENT_CHARGING
      during:
      %Begin Charging C22 Capacitor
      ATR_PACE_CTRL = LOW
      VENT_PACE_CTRL = LOW
      PACING_REF_PWM = VENT_DUTY_CYCLE
      PACE_CHARGE_CTRL = HIGH
      %Begin Discharging C21 Blocking Capacitor
      PACE_GND_CTRL = HIGH
      VENT_PACE_CTRL = LOW
      Z_ATR_CTRL = LOW
      Z_VENT_CTRL = LOW
      ATR_PACE_CTRL = LOW
      ATR_GND_CTRL = LOW
      VENT_GND_CTRL = HIGH
    state VENT_DISCHARGING
      during:
      %Discharge C22 into Ventricle (Vent Pacing)
      %Begin Charging Blocking Capacitor
      PACE_CHARGE_CTRL = LOW
      PACE_GND_CTRL = HIGH
      ATR_PACE_CTRL = LOW
      ATR_GND_CTRL = LOW
      Z_ATR_CTRL = LOW
      Z_VENT_CTRL = LOW
      VENT_GND_CTRL = LOW
      VENT_PACE_CTRL  = HIGH
    state ATR_CHARGING
      during:
      %Begin Charging C22 Capacitor
      ATR_PACE_CTRL = LOW
      VENT_PACE_CTRL = LOW
      PACING_REF_PWM = ATR_DUTY_CYCLE
      PACE_CHARGE_CTRL = HIGH
      %Begin Discharging C21 Blocking Capacitor
      PACE_GND_CTRL = HIGH
      VENT_PACE_CTRL = LOW
      Z_ATR_CTRL = LOW
      Z_VENT_CTRL = LOW
      ATR_PACE_CTRL = LOW
      ATR_GND_CTRL = HIGH
      VENT_GND_CTRL = LOW
    state ATR_DISCHARGING
      during:
      %Discharge C22 into Atrium (AtrialPacing)
      %Begin Charging C21 Blocking Capacitor
      PACE_CHARGE_CTRL = LOW
      PACE_GND_CTRL = HIGH
      ATR_PACE_CTRL = HIGH
      ATR_GND_CTRL = LOW
      Z_ATR_CTRL = LOW
      Z_VENT_CTRL = LOW
      VENT_GND_CTRL = LOW
      VENT_PACE_CTRL  = LOW
    VENT_DISCHARGING -> VENT_CHARGING : after(VENT_PW,msec)
    ATR_DISCHARGING -> ATR_CHARGING : after(ATR_PW, msec)
    ATR_CHARGING -> (junction 629)
    (junction 629) -> VENT_DISCHARGING [order 1] : after(MODULATED_PERIOD - AV_DELAY- ATR_PW,msec)
    VENT_CHARGING -> (junction 619) [order 1]
    (junction 619) -> ATR_DISCHARGING [order 2] : after(MODULATED_PERIOD - VENT_PW, msec)
    (junction 619) -> ATR_CHARGING [order 1] : [ATR_CMP_DETECT == HIGH ]
    (junction 629) -> VENT_CHARGING [order 2] : [VENT_CMP_DETECT == HIGH]
  Start -> VENT_CHARGING [order 9] : [MODE == 9]
  VVIR.CHARGING -> Start [order 3] : [MODE ~= 8]
  VENT_CHARGING -> Start [order 2] : [MODE ~= 9]
  Start -> VVIR.CHARGING [order 8] : [MODE == 8]
  Start -> CHARGE_AAIR [order 7] : [MODE == 7]
  Start -> VOOR.CHARGING [order 6] : [MODE == 6]
  Start -> AOOR.CHARGING [order 5] : [MODE == 5]
  Start -> VVI.CHARGING [order 3] : [MODE == 4]
  AOO.CHARGING -> Start [order 2] : [MODE ~= 1]
  AAI.CHARGING -> Start [order 3] : [MODE ~= 2]
  CHARGE_AAIR -> Start [order 3] : [MODE ~= 7]
  Start -> AOO.CHARGING [order 1] : [MODE == 1]
  VVI.CHARGING -> Start [order 3] : [MODE ~= 4]
  AOOR.CHARGING -> Start [order 2] : [MODE ~= 5]
  Start -> VOO.CHARGING [order 4] : [MODE == 3]
  Start -> AAI.CHARGING [order 2] : [MODE == 2]
  VOO.CHARGING -> Start [order 2] : [MODE ~= 3]
  VOOR.CHARGING -> Start [order 2] : [MODE ~= 6]
  (default) -> Start
  data: ATR_PACE_CTRL output boolean; ATR_GND_CTRL output boolean; Z_ATR_CTRL output boolean; VENT_PACE_CTRL output boolean; VENT_GND_CTRL output boolean; Z_VENT_CTRL output boolean; PACE_GND_CTRL output boolean; PACING_REF_PWM output double; LOWER_RATE_LIMIT input uint16; PERIOD input double; MODE input uint16; ATR_DUTY_CYCLE input double; ATR_PW input uint16; ARP input uint16; VENT_PW input uint16; VENT_DUTY_CYCLE input double; VRP input uint16; PACE_CHARGE_CTRL output boolean; HIGH local boolean =true; LOW local boolean =false; ATR_CMP_DETECT input boolean; VENT_CMP_DETECT input boolean; FRONTEND_CTRL output boolean =true; AV_DELAY input; MODULATED_PERIOD input; assignable local; Pace local

== stateflow chart allmodes_group11/Stateflow/Chart1 ==
  state S4
    entry:
    ADAPTED_RATE = ADAPTED_RATE + step_up;
  state S3
    entry:
    ADAPTED_RATE = TARGET_RATE;
  state Start1
    entry:
    ADAPTED_RATE = LOWER_RATE_LIMIT;
  state S_FAILSAFE1
    entry:
    ADAPTED_RATE = ADAPTED_RATE - step_up;
  state S2FAIL1
    entry:
    ADAPTED_RATE = ADAPTED_RATE - step_down;
  (default) -> Start1 : {step_up = ceil((MAX_SENSE - LOWER_RATE_LIMIT) / REACT_TIME),
      | step_down = ceil((MAX_SENSE - LOWER_RATE_LIMIT)  / RCVR_TIME)}
  S4 -> S4 [order 1] : after(1000,msec)[ADAPTED_RATE <= TARGET_RATE]
  S3 -> S3 [order 2] : [ACTIVITY > ACTIVITY_THRESH]
  S4 -> S3 [order 3] : [ADAPTED_RATE >= TARGET_RATE]
  Start1 -> S4 [order 1] : [ACTIVITY >= ACTIVITY_THRESH]
  Start1 -> Start1 [order 2] : [ACTIVITY < ACTIVITY_THRESH]
  S3 -> S2FAIL1 [order 1] : [ACTIVITY < ACTIVITY_THRESH]
  S4 -> S_FAILSAFE1 [order 2] : [ACTIVITY <  ACTIVITY_THRESH]
  S_FAILSAFE1 -> S4 [order 1] : [ACTIVITY >= ACTIVITY_THRESH]
  S2FAIL1 -> S4 [order 3] : [ACTIVITY >= ACTIVITY_THRESH]
  S2FAIL1 -> Start1 [order 1] : [ADAPTED_RATE <= LOWER_RATE_LIMIT]
  S_FAILSAFE1 -> S2FAIL1 [order 2] : [ after(1000,msec)]
  S2FAIL1 -> S2FAIL1 [order 2] : after(1000, msec)[ADAPTED_RATE >= LOWER_RATE_LIMIT]
  data: ACTIVITY input; ADAPTED_RATE output double; MAX_SENSE input double; REACT_TIME input double; RESP_FACTOR input double; ACTIVITY_THRESH input double; RCVR_TIME input double; LOWER_RATE_LIMIT input double; step_up local double; step_down local double; TARGET_RATE input double
